simulink model "experimen3_with_individual_thyristors"  (R2023a)
settings: Solver=VariableStepAuto  StartTime=0.0  StopTime=0.04  RelTol=1e-3
undefined symbols (not defined in the file): D1, Delta
libraries: spsThyristorLib x12, spsACVoltageSourceLib x3, spsCurrentMeasurementLib x1, spsGroundLib x1, spsSeriesRLCBranchLib x1, spsThreePhaseTransformerThreeWindingsLib x1, spsVoltageMeasurementLib x1, sps_lib x1
settings Model: Creator=hp 1  LastModifiedBy=hp 1

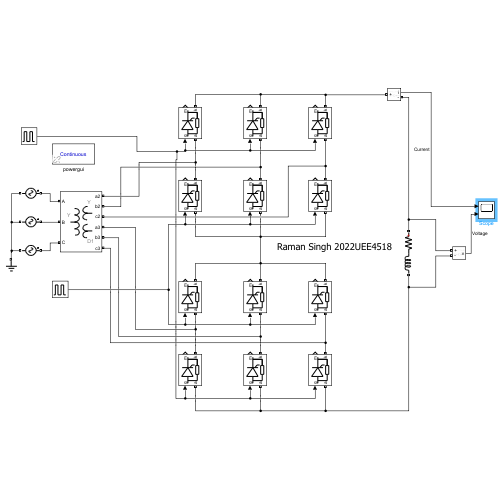
[thumbnail: Simulink's stored preview of the top-level diagram]
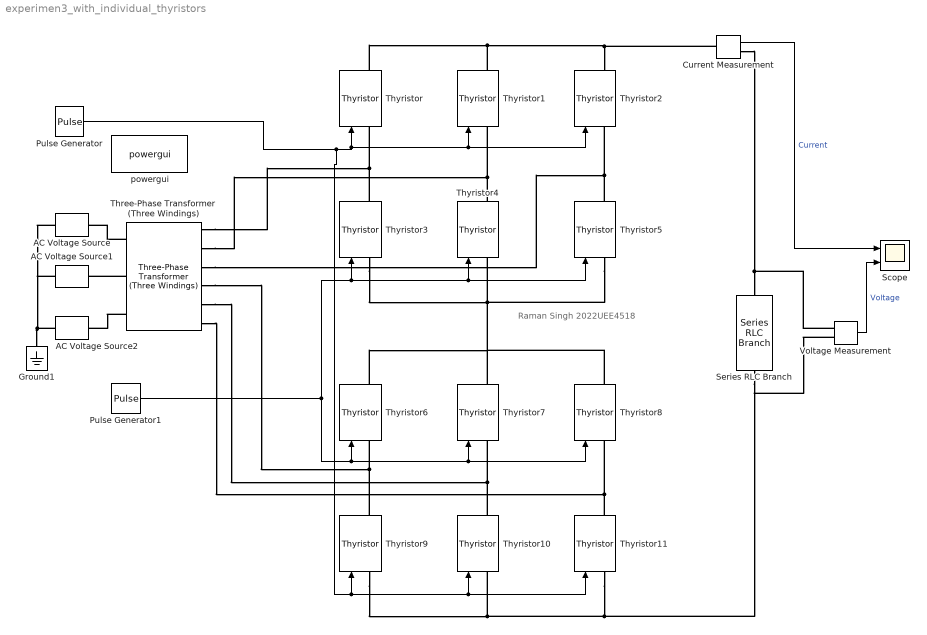
== system experimen3_with_individual_thyristors ==
  note: Raman Singh 2022UEE4518
  AC Voltage Source : spsACVoltageSourceLib/AC Voltage Source  Amplitude=240  Phase=0  Frequency=50  SampleTime=0  Measurements=None  BusType=swing  Pref=10e3  Qref=0  Qmin=-inf  Qmax=+inf
  AC Voltage Source1 : spsACVoltageSourceLib/AC Voltage Source  Amplitude=240  Phase=-120  Frequency=50  SampleTime=0  Measurements=None  BusType=swing  Pref=10e3  Qref=0  Qmin=-inf  Qmax=+inf
  AC Voltage Source2 : spsACVoltageSourceLib/AC Voltage Source  Amplitude=240  Phase=-240  Frequency=50  SampleTime=0  Measurements=None  BusType=swing  Pref=10e3  Qref=0  Qmin=-inf  Qmax=+inf
  Current Measurement : spsCurrentMeasurementLib/Current Measurement  PhasorSimulation=off  OutputType=Complex  PSBequivalent=0
  Ground1 : spsGroundLib/Ground  LConnTagsString=a
  Pulse Generator : DiscretePulseGenerator  PulseType=Time based  Period=10  PulseWidth=5
  Pulse Generator1 : DiscretePulseGenerator  PulseType=Time based  Period=10  PulseWidth=5
  Scope : Scope  NumInputPorts=2
  Series RLC Branch : spsSeriesRLCBranchLib/Series RLC Branch  LConnTagsString=__new0  RConnTagsString=__new0  BranchType=RL  Resistance=100  Inductance=0.25  SetiL0=off  InitialCurrent=0  Capacitance=1e-6  Setx0=off  InitialVoltage=0  Measurements=None
  Three-Phase Transformer (Three Windings) : spsThreePhaseTransformerThreeWindingsLib/Three-Phase Transformer (Three Windings)  Winding1Connection=Y  Winding2Connection=Y  Winding3Connection=Delta (D1)  CoreType=Three single-phase transformers  SetSaturation=off  Hysteresis=off  DataFile='hysteresis'  SetInitialFlux=off  Measurements=None  UNITS=pu  NominalPower=[ 250e6 , 50 ]  Winding1=[240 0.01 0.01 ]  Winding2=[240 0.01 0.01 ]  Winding3=[240 0.01 0.01 ]  Rm=500  Lm=500  L0=0.5  Saturation=[ 0,0 ; 0.0024,1.2 ; 1.0,1.52 ]  InitialFluxes=[0.8 -0.8 0.7]  BreakLoop=off  DiscreteSolver=Trapezoidal iterative  DataType=off  TransfoNumber=1
      settings: LibrarySourceBlock=|
      | sps_lib/Power Grid Elements/Three-Phase
      | Transformer
      | (Three Windings)
  Thyristor{,1..11} (12 alike) : spsThyristorLib/Thyristor  Ron=0.001  Lon=0  Vf=0.8  IC=0  Rs=500  Cs=250e-9  Measurements=on
  Voltage Measurement : spsVoltageMeasurementLib/Voltage Measurement  PhasorSimulation=off  OutputType=Complex  PSBequivalent=0
  powergui : sps_lib/powergui  Priority=1  SimulationMode=Continuous  SampleTime=50e-6  frequency=60  Iterations=50  frequencyindice=50  Pbase=100e6  ErrMax=1e-4  UnitsV=kV  UnitsW=MW  buscounter=0  FunctionMessages=off  echomessages=off  EnableUseOfTLC=off  CurrentSourceSwitches=off  DisableSnubberDevices=off  DisableRonSwitches=off  DisableVfSwitches=off  DisplayEquations=off  AutomaticDiscreteSolvers=off  SolverType=Tustin/Backward Euler (TBE)  Interpol=off  ExternalGateDelay=off  methode=off  Ts=100  x0status=blocks  SPID=on  SwTol=0  HookPort=off  NonlinearTolerance=1e-4  nMaxIteration=100  ContinueOnMaxIteration=off  RestoreLinks=warning  ResistiveCurrentMeasurement=off  Frange=[0:2:500]  Ylog=off  Xlog=on  ShowGrid=off  save=off  variable=ZData  structure=0  ZoomFFT=off  StartTime=0.0  cycles=1  DisplayStyle=1  fundamental=60  FreqAxis=off  MaxFrequency=1000  frequencyindicesteady=1  RmsSteady=1  display=off
  wires:
  Pulse Generator1/1 -> Thyristor8/1, Thyristor7/1, Thyristor6/1, Thyristor5/1, Thyristor4/1, Thyristor3/1
  Pulse Generator/1 -> Thyristor11/1, Thyristor10/1, Thyristor9/1, Thyristor2/1, Thyristor1/1, Thyristor/1
  Current Measurement/1 -> Scope/1  "Current"
  Voltage Measurement/1 -> Scope/2  "Voltage"
  connections:
  AC Voltage Source2/LConn1 -- AC Voltage Source/LConn1 -- AC Voltage Source1/LConn1 -- Ground1/LConn1
  Thyristor3/RConn1 -- Three-Phase Transformer (Three Windings)/RConn1 -- Thyristor/LConn1
  Thyristor4/RConn1 -- Three-Phase Transformer (Three Windings)/RConn2 -- Thyristor1/LConn1
  Thyristor5/RConn1 -- Three-Phase Transformer (Three Windings)/RConn3 -- Thyristor2/LConn1
  Thyristor/RConn1 -- Thyristor1/RConn1 -- Current Measurement/LConn1 -- Thyristor2/RConn1
  Thyristor3/LConn1 -- Thyristor8/RConn1 -- Thyristor6/RConn1 -- Thyristor7/RConn1 -- Thyristor5/LConn1 -- Thyristor4/LConn1
  Thyristor9/LConn1 -- Voltage Measurement/LConn2 -- Series RLC Branch/RConn1 -- Thyristor11/LConn1 -- Thyristor10/LConn1
  Thyristor10/RConn1 -- Three-Phase Transformer (Three Windings)/RConn5 -- Thyristor7/LConn1
  Thyristor9/RConn1 -- Three-Phase Transformer (Three Windings)/RConn4 -- Thyristor6/LConn1
  Thyristor11/RConn1 -- Three-Phase Transformer (Three Windings)/RConn6 -- Thyristor8/LConn1
  Three-Phase Transformer (Three Windings)/LConn1 -- AC Voltage Source/RConn1
  Three-Phase Transformer (Three Windings)/LConn2 -- AC Voltage Source1/RConn1
  Three-Phase Transformer (Three Windings)/LConn3 -- AC Voltage Source2/RConn1
  Current Measurement/RConn1 -- Voltage Measurement/LConn1 -- Series RLC Branch/LConn1
